simulink model "OSWEC"  (R2021b)
settings: Solver=ode45  StartTime=0  StopTime=200  FixedStep=0.01  MaxStep=0.01  RelTol=1e-3  EnableMultiTasking=on
values from neighbouring files (symbols this model uses):
  N = 25    [PI_reg_nocodesign.mat]
  ptosim = ptoSimClass('Non-Compressible Fluid Hydraulic')    [wecSimInputFile.m]
undefined symbols (not defined in the file or in its folder): body, constraint, geometry, hydroData, pto, X, Y, Z
libraries: nesl_utility x8, sm_lib x7, WECSim_Lib_Body_Elements x2, WECSim_Lib_Constraints x1, WECSim_Lib_Frames x1, PTOSim_Lib x1
settings Model: Creator=mlawson  LastModifiedBy=jackson
settings SolverCC: ZeroCrossControl=DisableAll  AlgebraicLoopSolver=LineSearch  AutoInsertRateTranBlk=on
settings DataIOCC: SaveFormat=Array  SaveOutput=off  SaveTime=off  ReturnWorkspaceOutputs=off
settings OptimizationCC: LifeSpan=inf  SimCompilerOptimization=on
settings DebuggingCC: UnderspecifiedInitializationDetection=Classic  MergeDetectMultiDrivingBlocksExec=none  SolverPrmCheckMsg=warning  AllowSymbolicDim=off  StateNameClashWarn=warning  SFUnexpectedBacktrackingDiag=warning  SFNoUnconditionalDefaultTransitionDiag=warning  SFExecutionAtInitializationDiag=none  SFMachineParentedDataDiag=warning  ArithmeticOperatorsInVariantConditions=warning
settings HardwareCC: ProdBitPerPointer=32  ProdBitPerSizeT=32  ProdBitPerPtrDiffT=32  ProdLargestAtomicFloat=None  ProdIntDivRoundTo=Undefined  ProdEndianess=Unspecified  ProdWordSize=32  ProdHWDeviceType=32-bit Generic
settings ModelReferenceCC: PropagateSignalLabelsOutOfModel=off
settings SFSimCC: SimUseLocalCustomCode=off  CustomCodeUndefinedFunction=UseInterfaceOnly
settings RTWCC: RTWUseLocalCustomCode=off
settings CodeAppCC: StateflowObjectComments=on
settings GRTTargetCC: TargetLangStandard=C89/C90 (ANSI)
settings ConfigComp: CovMetricSettings=dw  CovSaveCumulativeToWorkspaceVar=on  CovSaveSingleToWorkspaceVar=on  CovExternalEMLEnable=off  CovSFcnEnable=off
settings SimscapeCC: SimscapeNormalizeSystem=off
settings ConfigurationSet: Description=SimMechanics 2G
settings ExplorerConfigSet: SimMechanicsOpenEditorOnUpdate=off  InternalSimMechanicsExplorerSettings="<ExplorerConfiguration><canonicalview>default</canonicalview><TilePanel><TileInfo><Tiles Columns=\"1\" Count=\"1\" Rows=\"1\"><Column Left=\"2\" Weight=\"1\"/><Column Left=\"1335\"/><Row Top=\"2\" Weight=\"1\"/><Row Top=\"911\"/><Tile Height=\"1\" Width=\"1\" X=\"0\" Y=\"0\"/></Tiles></TileInfo><SceneInfo><SceneViewer><BGColor><R>0.60000002384185791</R><G>0.60000002384185791</G><B>0.60000002384185791</B></BGColor><Camera><Position><X>365.37645888990272</X><Y>-369.82486814446582</Y><Z>359.64809521743916</Z></Position><Center><X>-6.7351450971904585</X><Y>2.2867358426280204</Y><Z>-12.463508769654169</Z></Center><Up><X>-0.40824829046386307</X><Y>0.40824829046386307</Y><Z>0.81649658092772615</Z></Up><Left>-57.820127362122818</Left><Right>57.820127362122818</Right><Bottom>-38.308817187253304</Bottom><Top>38.308817187253304</Top></Camera></SceneViewer></SceneInfo></TilePanel></ExplorerConfiguration>"

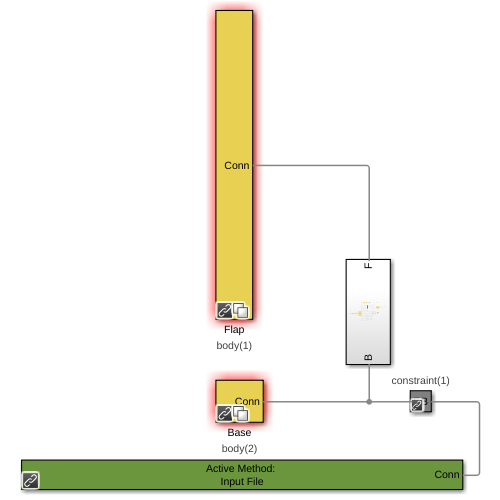
[thumbnail: Simulink's stored preview of the top-level diagram]
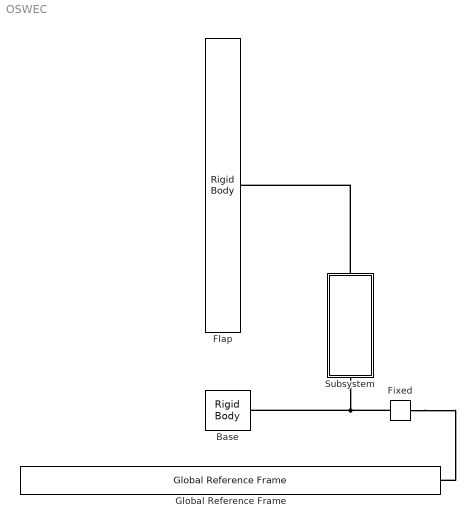
== system OSWEC ==
  Base : WECSim_Lib_Body_Elements/Rigid Body  body=body(2)  h5File=hydroData/*.h5  geometryFile=geometry/*.stl  mass=0  momOfInertia=0 0 0  nhBody=0  nlHydro=0  cg=0 0 0  cb=0 0 0  dof=6  dispVol=0  initLinDisp=0 0 0  initAngularDispAxis=0 1 0  initAngularDispAngle=0  option=0  cd=0 0 0  ca=0 0 0  characteristicArea=0 0 0  VME=0  rgME=0 0 0  z=0 0 1
      settings: SourceProductName=WEC-Sim
  Fixed : WECSim_Lib_Constraints/Fixed  constraint=constraint(1)  loc="0  0  0"  initLinDisp=0 0 0  y=0 1 0  z=0 0 1  upperLimitSpecify=off  upperLimitBound=0  upperLimitTransitionRegionWidth=0  upperLimitStiffness=0  upperLimitDamping=0  lowerLimitSpecify=off  lowerLimitBound=0  lowerLimitTransitionRegionWidth=0  lowerLimitStiffness=0  lowerLimitDamping=0
      settings: AttributesFormatString=%<constraint>  SourceProductName=WEC-Sim
  Flap : WECSim_Lib_Body_Elements/Rigid Body  body=body(1)  h5File=hydroData/*.h5  geometryFile=geometry/*.stl  mass=0  momOfInertia=0 0 0  nhBody=0  nlHydro=0  cg=0 0 0  cb=0 0 0  dof=6  dispVol=0  initLinDisp=0 0 0  initAngularDispAxis=0 1 0  initAngularDispAngle=0  option=0  cd=0 0 0  ca=0 0 0  characteristicArea=0 0 0  VME=0  rgME=0 0 0  z=0 0 1
      settings: SourceProductName=WEC-Sim
  Global Reference Frame : WECSim_Lib_Frames/Global Reference Frame  waves=waves  simu=simu  ParamInput=Input File  InputFile=wecSimInputFile.m  mode=normal  explorer=off  solver=ode4  startTime=0  rampTime=100  endTime=400  dt=0.1  CITime=60  ssCalc=0  WaveClass=regular  H=2.5  T=8  etaDataFile=NOT DEFINED  spectrumDataFile=NOT DEFINED  waveDir=0  waveSpread=1  spectrumType=NOT DEFINED  freqDisc=EqualEnergy  phaseSeed=0
      settings: SourceProductName=WEC-Sim
  Subsystem : Subsystem
  connections:
  Fixed/LConn1 -- Global Reference Frame/RConn1
  Fixed/RConn1 -- Base/RConn1 -- Subsystem/LConn1
  Subsystem/RConn1 -- Flap/RConn1

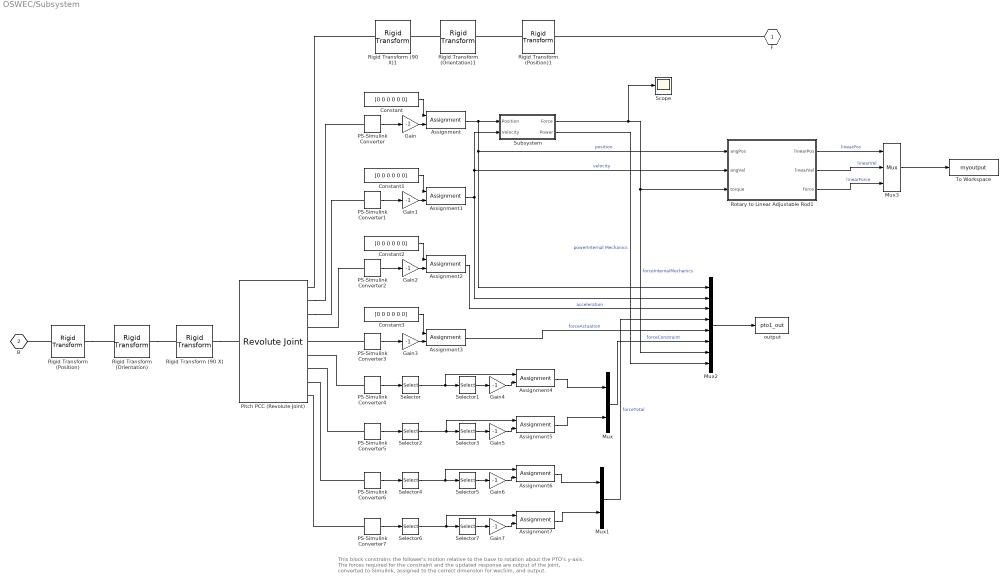
== system OSWEC/Subsystem ==
  note: This block constrains the follower's motion relative to the base to rotation about the PTO's y-axis. The forces required for the constraint and the updated response are output of the joint, converted to Simulink, assigned to the correct dimension for wecSim, and output.
  "Assignment " : Assignment  IndexOptions=Index vector (dialog)  Indices=5  OutputSizes=1
  Assignment1 : Assignment  IndexOptions=Index vector (dialog)  Indices=5  OutputSizes=1
  Assignment2 : Assignment  IndexOptions=Index vector (dialog)  Indices=5  OutputSizes=1
  Assignment3 : Assignment  IndexOptions=Index vector (dialog)  Indices=5  OutputSizes=1
  Assignment{4..7} (4 alike) : Assignment  DiagnosticForDimensions=Warning  IndexOptions=Index vector (dialog)  Indices=2  OutputSizes=1
  Constant{,1..3} (4 alike) : Constant  Value=[0 0 0 0 0 0]
  Gain{,1..7} (8 alike) : Gain  Gain=-1
  Mux : Mux  Inputs=2
  Mux1 : Mux  Inputs=2
  Mux2 : Mux  Inputs=8
  Mux3 : Mux  Inputs=3
  PS-Simulink Converter{,1..7} (8 alike) : nesl_utility/PS-Simulink Converter  PhysicalDomain=network_engine_domain  SubClassName=ps_output  LeftPortType=input  RightPortType=output  PseudoPeriodic=off  Frequencies=[]  Unit=1  AffineConversion=off
      settings: SourceProductBaseCode=PW,SS
  Pitch PCC (Revolute Joint) : sm_lib/Joints/Revolute Joint  JointMode=Normal  SenseConstraintForce=on  SenseConstraintForceX=off  SenseConstraintForceY=off  SenseConstraintForceZ=off  SenseConstraintTorque=on  SenseConstraintTorqueX=off  SenseConstraintTorqueY=off  SenseConstraintTorqueZ=off  SenseTotalForce=on  SenseTotalForceX=off  SenseTotalForceY=off  SenseTotalForceZ=off  SenseTotalTorque=on  SenseTotalTorqueX=off  SenseTotalTorqueY=off  SenseTotalTorqueZ=off  CompositeWrenchDir=BaseOnFollower  CompositeWrenchFrame=BaseFrame  EquilibriumPosition=pto.equilibriumPosition  EquilibriumPositionUnits=deg  SpringStiffness=pto.k  SpringStiffnessUnits=N*m/rad  DampingCoefficient=pto.c  DampingCoefficientUnits=N*m/(rad/s)  TorqueActuationMode=NoTorque  MotionActuationMode=ComputedMotion  SensePosition=on  SenseVelocity=on  SenseAcceleration=on  SenseTorqueForce=on  SenseLowerLimitTorqueForce=off  SenseUpperLimitTorqueForce=off  LowerLimitSpecify=off  LowerLimitBound=pto.hardStops.lowerLimitBound  LowerLimitBoundUnits=deg  LowerLimitStiffness=pto.hardStops.lowerLimitStiffness  LowerLimitStiffnessUnits=N*m/deg  LowerLimitDamping=pto.hardStops.lowerLimitDamping  LowerLimitDampingUnits=N*m/(deg/s)  LowerLimitTransitionRegionWidth=pto.hardStops.lowerLimitTransitionRegionWidth  LowerLimitTransitionRegionWidthUnits=deg  UpperLimitSpecify=off  UpperLimitBound=pto.hardStops.upperLimitBound  UpperLimitBoundUnits=deg  UpperLimitStiffness=pto.hardStops.upperLimitStiffness  UpperLimitStiffnessUnits=N*m/deg  UpperLimitDamping=pto.hardStops.upperLimitDamping  UpperLimitDampingUnits=N*m/(deg/s)  UpperLimitTransitionRegionWidth=pto.hardStops.upperLimitTransitionRegionWidth  UpperLimitTransitionRegionWidthUnits=deg  PositionTargetSpecify=off  PositionTargetPriority=High  PositionTargetValue=0  PositionTargetValueUnits=deg  VelocityTargetSpecify=off  VelocityTargetPriority=High  VelocityTargetValue=0  VelocityTargetValueUnits=deg/s
  Rigid Transform (Position) : sm_lib/Frames and Transforms/Rigid Transform  TranslationMethod=Cartesian  TranslationStandardOffset=0  TranslationLengthUnit=m  TranslationStandardAxis=+Z  TranslationCartesianOffset=pto.initDisp.initLinDisp + pto.loc  TranslationROffset=0  TranslationROffsetUnits=m  TranslationZOffset=0  TranslationZOffsetUnits=m  TranslationThetaOffset=0  TranslationThetaOffsetUnits=deg  RotationMethod=None  RotationAngleUnits=rad  RotationStandardAxis=+Y  RotationAngle=0  RotationArbitraryAxis=[0 1 0]  FollAlignAxisA=+X  BaseAlignAxisA=+Y  FollAlignAxisB=+Y  BaseAlignAxisB=+Z  RotationSequenceAxes=FollowerAxes  RotationSequence=XYX  RotationSequenceAngles=[0 0 0]  RotationSequenceAnglesUnits=deg  RotationMatrix=[1 0 0; 0 1 0; 0 0 1]
  Rigid Transform (Position)1 : sm_lib/Frames and Transforms/Rigid Transform  TranslationMethod=Cartesian  TranslationStandardOffset=0  TranslationLengthUnit=m  TranslationStandardAxis=+Z  TranslationCartesianOffset=pto.initDisp.initLinDisp + pto.loc  TranslationROffset=0  TranslationROffsetUnits=m  TranslationZOffset=0  TranslationZOffsetUnits=m  TranslationThetaOffset=0  TranslationThetaOffsetUnits=deg  RotationMethod=None  RotationAngleUnits=rad  RotationStandardAxis=+Y  RotationAngle=0  RotationArbitraryAxis=[0 1 0]  FollAlignAxisA=+X  BaseAlignAxisA=+Y  FollAlignAxisB=+Y  BaseAlignAxisB=+Z  RotationSequenceAxes=FollowerAxes  RotationSequence=XYX  RotationSequenceAngles=[0 0 0]  RotationSequenceAnglesUnits=deg  RotationMatrix=[1 0 0; 0 1 0; 0 0 1]
  Rigid Transform (90 X) : sm_lib/Frames and Transforms/Rigid Transform  TranslationMethod=None  TranslationStandardOffset=0  TranslationLengthUnit=m  TranslationStandardAxis=+Z  TranslationCartesianOffset=0  TranslationROffset=0  TranslationROffsetUnits=m  TranslationZOffset=0  TranslationZOffsetUnits=m  TranslationThetaOffset=0  TranslationThetaOffsetUnits=deg  RotationMethod=StandardAxis  RotationAngleUnits=deg  RotationStandardAxis=+X  RotationAngle=90  RotationArbitraryAxis=[0 1 0]  FollAlignAxisA=+X  BaseAlignAxisA=+Y  FollAlignAxisB=+Y  BaseAlignAxisB=+Z  RotationSequenceAxes=FollowerAxes  RotationSequence=XYX  RotationSequenceAngles=[0 0 0]  RotationSequenceAnglesUnits=deg  RotationMatrix=[1 0 0; 0 1 0; 0 0 1]
  Rigid Transform (90 X)1 : sm_lib/Frames and Transforms/Rigid Transform  TranslationMethod=None  TranslationStandardOffset=0  TranslationLengthUnit=m  TranslationStandardAxis=+Z  TranslationCartesianOffset=0  TranslationROffset=0  TranslationROffsetUnits=m  TranslationZOffset=0  TranslationZOffsetUnits=m  TranslationThetaOffset=0  TranslationThetaOffsetUnits=deg  RotationMethod=StandardAxis  RotationAngleUnits=deg  RotationStandardAxis=+X  RotationAngle=90  RotationArbitraryAxis=[0 1 0]  FollAlignAxisA=+X  BaseAlignAxisA=+Y  FollAlignAxisB=+Y  BaseAlignAxisB=+Z  RotationSequenceAxes=FollowerAxes  RotationSequence=XYX  RotationSequenceAngles=[0 0 0]  RotationSequenceAnglesUnits=deg  RotationMatrix=[1 0 0; 0 1 0; 0 0 1]
  Rigid Transform (Orientation) : sm_lib/Frames and Transforms/Rigid Transform  TranslationMethod=None  TranslationStandardOffset=0  TranslationLengthUnit=m  TranslationStandardAxis=+Z  TranslationCartesianOffset=0  TranslationROffset=0  TranslationROffsetUnits=m  TranslationZOffset=0  TranslationZOffsetUnits=m  TranslationThetaOffset=0  TranslationThetaOffsetUnits=deg  RotationMethod=RotationMatrix  RotationAngleUnits=rad  RotationStandardAxis=+Y  RotationAngle=0  RotationArbitraryAxis=[0 1 0]  FollAlignAxisA=+X  BaseAlignAxisA=+Y  FollAlignAxisB=+Y  BaseAlignAxisB=+Z  RotationSequenceAxes=FollowerAxes  RotationSequence=XYX  RotationSequenceAngles=[0 0 0]  RotationSequenceAnglesUnits=deg  RotationMatrix=pto.orientation.rotationMatrix
  Rigid Transform (Orientation)1 : sm_lib/Frames and Transforms/Rigid Transform  TranslationMethod=None  TranslationStandardOffset=0  TranslationLengthUnit=m  TranslationStandardAxis=+Z  TranslationCartesianOffset=0  TranslationROffset=0  TranslationROffsetUnits=m  TranslationZOffset=0  TranslationZOffsetUnits=m  TranslationThetaOffset=0  TranslationThetaOffsetUnits=deg  RotationMethod=RotationMatrix  RotationAngleUnits=rad  RotationStandardAxis=+Y  RotationAngle=0  RotationArbitraryAxis=[0 1 0]  FollAlignAxisA=+X  BaseAlignAxisA=+Y  FollAlignAxisB=+Y  BaseAlignAxisB=+Z  RotationSequenceAxes=FollowerAxes  RotationSequence=XYX  RotationSequenceAngles=[0 0 0]  RotationSequenceAnglesUnits=deg  RotationMatrix=pto.orientation.rotationMatrix
  Rotary to Linear Adjustable Rod1 : Subsystem  AncestorBlock=PTOSim_Lib/Motion Conversion/Rotary to Linear Adjustable Rod  mask{ptosim=ptosim.motionMechanism(1)}
      mask prompts: ptosim "Telescope Name:"
      mask init:
      | % if exist('ptosim','var')
      | %     h = [gcb '/To Workspace'];
      | %     responseName = ['motionMechanism' num2str(ptosim.number) '_out'];
      | %     set_param(h,'VariableName',responseName);
      | %     if ischar(ptosim.crank)==1 ...
      | %             || ischar(ptosim.rodInit)==1 ...
      | %             || ischar(ptosim.offset)==1 ...
      | %             error('One of the rotary to linear adjustable rod variables is undefined. For example, ptosim.motionMechanism.variableName')
      | %     end
      | % end
      | % clear h responseName
  Scope : Scope
  Selector{,2,4,6} (4 alike) : Selector  InputPortWidth=3  IndexOptions=Index vector (dialog)  Indices=[1 3 2]  OutputSizes=1
  Selector{1,3,5,7} (4 alike) : Selector  InputPortWidth=3  IndexOptions=Index vector (dialog)  Indices=[2]  OutputSizes=1
  Subsystem : Subsystem
  To Workspace : ToWorkspace  VariableName=myoutput  SaveFormat=Structure With Time  SampleTime=-1
  output : ToWorkspace  VariableName=pto1_out  SaveFormat=Structure With Time  SampleTime=-1
      settings: Decimation=round(simu.dtOut/simu.dt,0)
  F : PMIOPort  Side=Right
  B : PMIOPort  Port=2  Side=Left
  wires:
  Selector6/1 -> Selector7/1, Assignment7/1
  Gain4/1 -> Assignment4/2
  Selector2/1 -> Assignment5/1, Selector3/1
  Constant2/1 -> Assignment2/1
  PS-Simulink Converter3/1 -> Gain3/1
  Gain6/1 -> Assignment6/2
  Mux1/1 -> Mux2/4  "forceTotal"
  Assignment2/1 -> Mux2/3  "acceleration"
  Assignment3/1 -> Mux2/5  "forceActuation"
  Gain7/1 -> Assignment7/2
  Selector1/1 -> Gain4/1
  Gain3/1 -> Assignment3/2
  Gain/1 -> "Assignment "/2
  Selector7/1 -> Gain7/1
  PS-Simulink Converter/1 -> Gain/1
  Gain5/1 -> Assignment5/2
  Assignment6/1 -> Mux1/1
  Subsystem/2(Power) -> Mux2/8  "powerInternal Mechanics"
  Assignment7/1 -> Mux1/2
  PS-Simulink Converter6/1 -> Selector4/1
  Assignment1/1 -> Mux2/2, Subsystem/2(Velocity), Rotary to Linear Adjustable Rod1/2(angVel)  "velocity"
  Gain2/1 -> Assignment2/2
  Subsystem/1(Force) -> Scope/1, Rotary to Linear Adjustable Rod1/3(torque), Mux2/7  "forceInternalMechanics"
  Constant3/1 -> Assignment3/1
  PS-Simulink Converter7/1 -> Selector6/1
  Mux2/1 -> output/1
  PS-Simulink Converter4/1 -> Selector/1
  Gain1/1 -> Assignment1/2
  Selector5/1 -> Gain6/1
  Mux/1 -> Mux2/6  "forceConstraint"
  Constant1/1 -> Assignment1/1
  Assignment4/1 -> Mux/1
  "Assignment "/1 -> Rotary to Linear Adjustable Rod1/1(angPos), Mux2/1, Subsystem/1(Position)  "position"
  Selector4/1 -> Selector5/1, Assignment6/1
  PS-Simulink Converter1/1 -> Gain1/1
  Assignment5/1 -> Mux/2
  PS-Simulink Converter5/1 -> Selector2/1
  Selector3/1 -> Gain5/1
  PS-Simulink Converter2/1 -> Gain2/1
  Selector/1 -> Assignment4/1, Selector1/1
  Constant/1 -> "Assignment "/1
  Rotary to Linear Adjustable Rod1/1(linearPos) -> Mux3/1  "linearPos"
  Rotary to Linear Adjustable Rod1/2(linearVel) -> Mux3/2  "linearVel"
  Rotary to Linear Adjustable Rod1/3(force) -> Mux3/3  "linearForce"
  Mux3/1 -> To Workspace/1
  connections:
  Rigid Transform (Orientation)1/RConn1 -- Rigid Transform (90 X)1/LConn1
  PS-Simulink Converter5/LConn1 -- Pitch PCC (Revolute Joint)/RConn7
  Rigid Transform (Position)1/RConn1 -- Rigid Transform (Orientation)1/LConn1
  PS-Simulink Converter7/LConn1 -- Pitch PCC (Revolute Joint)/RConn9
  F/RConn1 -- Rigid Transform (Position)1/LConn1
  Pitch PCC (Revolute Joint)/RConn2 -- PS-Simulink Converter/LConn1
  PS-Simulink Converter4/LConn1 -- Pitch PCC (Revolute Joint)/RConn6
  PS-Simulink Converter6/LConn1 -- Pitch PCC (Revolute Joint)/RConn8
  Rigid Transform (Position)/RConn1 -- Rigid Transform (Orientation)/LConn1
  Rigid Transform (Orientation)/RConn1 -- Rigid Transform (90 X)/LConn1
  PS-Simulink Converter3/LConn1 -- Pitch PCC (Revolute Joint)/RConn5
  Rigid Transform (Position)/LConn1 -- B/RConn1
  PS-Simulink Converter2/LConn1 -- Pitch PCC (Revolute Joint)/RConn4
  Rigid Transform (90 X)1/RConn1 -- Pitch PCC (Revolute Joint)/RConn1
  Rigid Transform (90 X)/RConn1 -- Pitch PCC (Revolute Joint)/LConn1
  Pitch PCC (Revolute Joint)/RConn3 -- PS-Simulink Converter1/LConn1

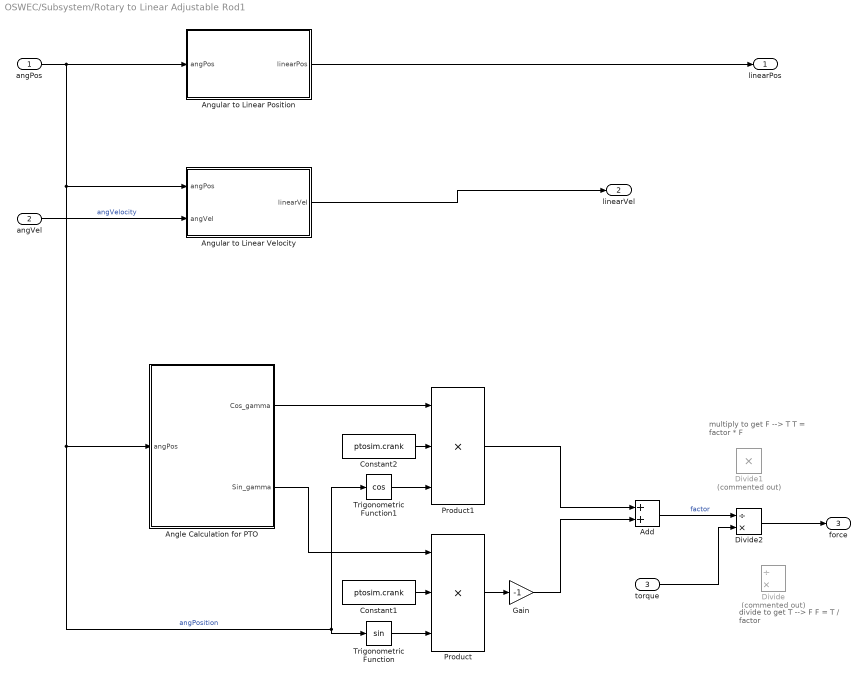
== system OSWEC/Subsystem/Rotary to Linear Adjustable Rod1 ==
  note: multiply to get F --> T
      | T = factor * F
  note: divide to get T --> F
      | F = T / factor
  angPos : Inport
  angVel : Inport  Port=2
  torque : Inport  Port=3
  Add : Sum
  Angle Calculation for PTO : Subsystem
  Angular to Linear Position : Subsystem
  Angular to Linear Velocity : Subsystem
  Constant1 : Constant  Value=ptosim.crank
  Constant2 : Constant  Value=ptosim.crank
  Divide : Product  Commented=on  Inputs=/*
  Divide1 : Product  Commented=on  Inputs=**
  Divide2 : Product  Inputs=/*
  Gain : Gain  Gain=-1
  Product : Product  Inputs=3
  Product1 : Product  Inputs=3
  Trigonometric Function : Trigonometry
  Trigonometric Function1 : Trigonometry  Operator=cos
  linearPos : Outport
  linearVel : Outport  Port=2
  force : Outport  Port=3
  wires:
  Product/1 -> Gain/1
  Constant1/1 -> Product/2
  Trigonometric Function/1 -> Product/3
  Constant2/1 -> Product1/2
  Angle Calculation for PTO/1(Cos_gamma) -> Product1/1
  Trigonometric Function1/1 -> Product1/3
  Angle Calculation for PTO/2(Sin_gamma) -> Product/1
  Gain/1 -> Add/2
  Product1/1 -> Add/1
  angPos/1 -> Angular to Linear Position/1(angPos), Trigonometric Function1/1, Trigonometric Function/1, Angle Calculation for PTO/1(angPos), Angular to Linear Velocity/1(angPos)  "angPosition"
  Angular to Linear Velocity/1(linearVel) -> linearVel/1
  angVel/1 -> Angular to Linear Velocity/2(angVel)  "angVelocity"
  Angular to Linear Position/1(linearPos) -> linearPos/1
  Divide2/1 -> force/1
  Add/1 -> Divide2/1  "factor"
  torque/1 -> Divide2/2

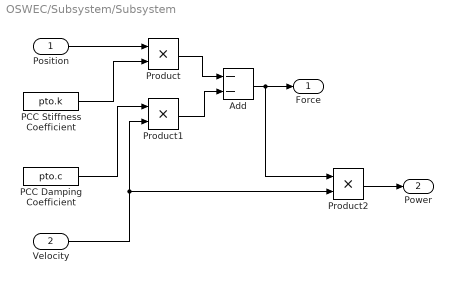
== system OSWEC/Subsystem/Subsystem ==
  Position : Inport
  Velocity : Inport  Port=2
  Add : Sum  Inputs=--
  PCC Damping Coefficient : Constant  Value=pto.c
  PCC Stiffness Coefficient : Constant  Value=pto.k
  Product : Product  Inputs=**
  Product1 : Product  Inputs=**
  Product2 : Product  Inputs=**
  Force : Outport
  Power : Outport  Port=2
  wires:
  PCC Damping Coefficient/1 -> Product1/1
  Velocity/1 -> Product2/2, Product1/2
  Position/1 -> Product/1
  Product2/1 -> Power/1
  PCC Stiffness Coefficient/1 -> Product/2
  Product/1 -> Add/1
  Product1/1 -> Add/2
  Add/1 -> Product2/1, Force/1

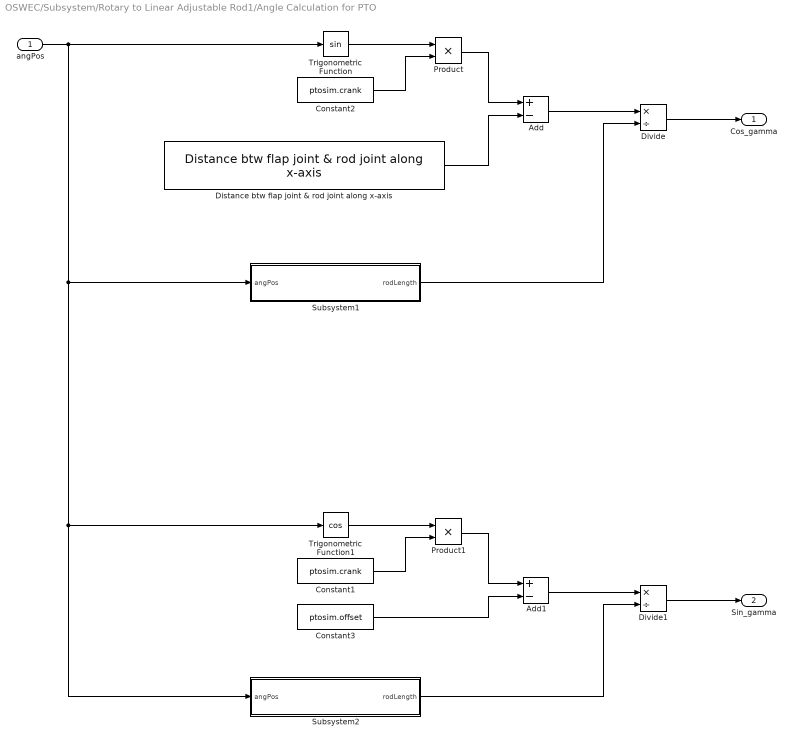
== system OSWEC/Subsystem/Rotary to Linear Adjustable Rod1/Angle Calculation for PTO ==
  angPos : Inport
  Add : Sum  Inputs=+-
  Add1 : Sum  Inputs=+-
  Constant1 : Constant  Value=ptosim.crank
  Constant2 : Constant  Value=ptosim.crank
  Constant3 : Constant  Value=ptosim.offset
  Distance btw flap joint & rod joint along x-axis : PTOSim_Lib/Motion Conversion/Rotary to Linear Adjustable Rod/Angular to Linear Velocity/Subsystem/Distance btw flap joint & rod joint along x-axis  SystemSampleTime=-1  VariantActivationTime=update diagram  Latency=0  AutoFrameSizeCalculation=off
      settings: SourceProductName=PTO-Sim
  Divide : Product  Inputs=*/
  Divide1 : Product  Inputs=*/
  Product : Product
  Product1 : Product
  Subsystem1 : Subsystem  AncestorBlock=|
      | PTOSim_Lib/Motion Conversion/Rotary to Linear
      | Adjustable Rod/Angular to Linear
      | Velocity/Subsystem
  Subsystem2 : Subsystem  AncestorBlock=|
      | PTOSim_Lib/Motion Conversion/Rotary to Linear
      | Adjustable Rod/Angular to Linear
      | Velocity/Subsystem
  Trigonometric Function : Trigonometry
  Trigonometric Function1 : Trigonometry  Operator=cos
  Cos_gamma : Outport
  Sin_gamma : Outport  Port=2
  wires:
  Divide1/1 -> Sin_gamma/1
  angPos/1 -> Trigonometric Function/1, Trigonometric Function1/1, Subsystem2/1(angPos), Subsystem1/1(angPos)
  Add1/1 -> Divide1/1
  Constant3/1 -> Add1/2
  Product1/1 -> Add1/1
  Constant1/1 -> Product1/2
  Trigonometric Function1/1 -> Product1/1
  Subsystem2/1(rodLength) -> Divide1/2
  Divide/1 -> Cos_gamma/1
  Subsystem1/1(rodLength) -> Divide/2
  Add/1 -> Divide/1
  Constant2/1 -> Product/2
  Distance btw flap joint & rod joint along x-axis/1 -> Add/2
  Product/1 -> Add/1
  Trigonometric Function/1 -> Product/1

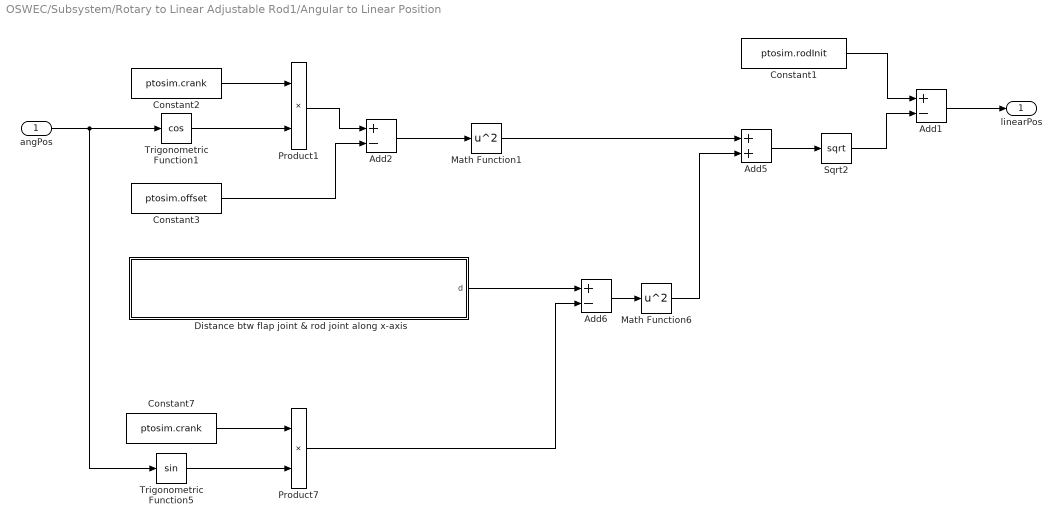
== system OSWEC/Subsystem/Rotary to Linear Adjustable Rod1/Angular to Linear Position ==
  angPos : Inport
  Add1 : Sum  Inputs=+-
  Add2 : Sum  Inputs=+-
  Add5 : Sum
  Add6 : Sum  Inputs=+-
  Constant1 : Constant  Value=ptosim.rodInit
  Constant2 : Constant  Value=ptosim.crank
  Constant3 : Constant  Value=ptosim.offset
  Constant7 : Constant  Value=ptosim.crank
  Distance btw flap joint & rod joint along x-axis : Subsystem
  Math Function1 : Math  Operator=square  SignedPower=on  SaturateOnIntegerOverflow=on
  Math Function6 : Math  Operator=square  SignedPower=on  SaturateOnIntegerOverflow=on
  Product1 : Product  Inputs=**
  Product7 : Product  Inputs=**
  Sqrt2 : Sqrt  SaturateOnIntegerOverflow=on
  Trigonometric Function1 : Trigonometry  Operator=cos
  Trigonometric Function5 : Trigonometry
  linearPos : Outport
  wires:
  Distance btw flap joint & rod joint along x-axis/1(d) -> Add6/1
  Constant7/1 -> Product7/1
  Math Function1/1 -> Add5/1
  Constant3/1 -> Add2/2
  Product1/1 -> Add2/1
  Trigonometric Function1/1 -> Product1/2
  Constant2/1 -> Product1/1
  Constant1/1 -> Add1/1
  Sqrt2/1 -> Add1/2
  Add5/1 -> Sqrt2/1
  Math Function6/1 -> Add5/2
  Add6/1 -> Math Function6/1
  Product7/1 -> Add6/2
  Trigonometric Function5/1 -> Product7/2
  Add2/1 -> Math Function1/1
  Add1/1 -> linearPos/1
  angPos/1 -> Trigonometric Function1/1, Trigonometric Function5/1

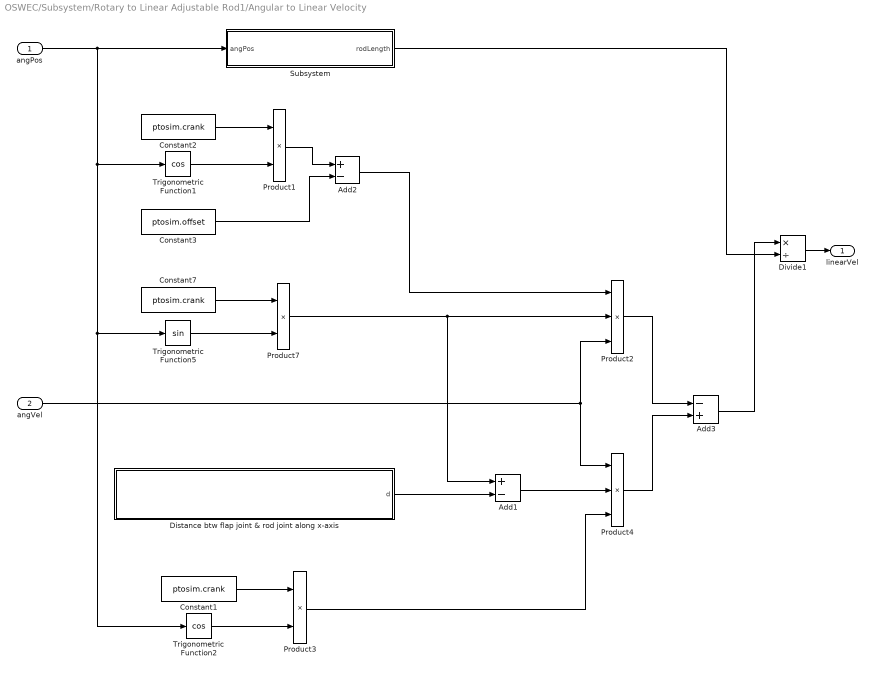
== system OSWEC/Subsystem/Rotary to Linear Adjustable Rod1/Angular to Linear Velocity ==
  angPos : Inport
  angVel : Inport  Port=2
  Add1 : Sum  Inputs=+-
  Add2 : Sum  Inputs=+-
  Add3 : Sum  Inputs=-+
  Constant1 : Constant  Value=ptosim.crank
  Constant2 : Constant  Value=ptosim.crank
  Constant3 : Constant  Value=ptosim.offset
  Constant7 : Constant  Value=ptosim.crank
  Distance btw flap joint & rod joint along x-axis : Subsystem
  Divide1 : Product  Inputs=*/
  Product1 : Product  Inputs=**
  Product2 : Product  Inputs=***
  Product3 : Product  Inputs=**
  Product4 : Product  Inputs=***
  Product7 : Product  Inputs=**
  Subsystem : Subsystem
  Trigonometric Function1 : Trigonometry  Operator=cos
  Trigonometric Function2 : Trigonometry  Operator=cos
  Trigonometric Function5 : Trigonometry
  linearVel : Outport
  wires:
  Divide1/1 -> linearVel/1
  Add3/1 -> Divide1/1
  Product4/1 -> Add3/2
  Product2/1 -> Add3/1
  Subsystem/1(rodLength) -> Divide1/2
  Add1/1 -> Product4/2
  angPos/1 -> Subsystem/1(angPos), Trigonometric Function1/1, Trigonometric Function2/1, Trigonometric Function5/1
  Product3/1 -> Product4/3
  Trigonometric Function2/1 -> Product3/2
  Constant1/1 -> Product3/1
  Distance btw flap joint & rod joint along x-axis/1(d) -> Add1/2
  angVel/1 -> Product4/1, Product2/3
  Constant7/1 -> Product7/1
  Product7/1 -> Product2/2, Add1/1
  Trigonometric Function5/1 -> Product7/2
  Constant3/1 -> Add2/2
  Product1/1 -> Add2/1
  Trigonometric Function1/1 -> Product1/2
  Constant2/1 -> Product1/1
  Add2/1 -> Product2/1

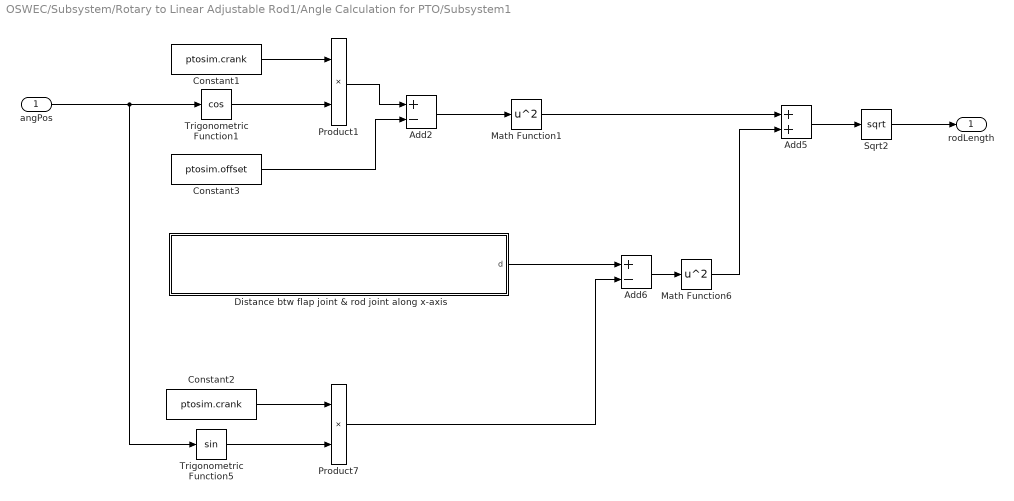
== system OSWEC/Subsystem/Rotary to Linear Adjustable Rod1/Angle Calculation for PTO/Subsystem1 ==
  angPos : Inport
  Add2 : Sum  Inputs=+-
  Add5 : Sum
  Add6 : Sum  Inputs=+-
  Constant1 : Constant  Value=ptosim.crank
  Constant2 : Constant  Value=ptosim.crank
  Constant3 : Constant  Value=ptosim.offset
  Distance btw flap joint & rod joint along x-axis : Subsystem
  Math Function1 : Math  Operator=square  SignedPower=on  SaturateOnIntegerOverflow=on
  Math Function6 : Math  Operator=square  SignedPower=on  SaturateOnIntegerOverflow=on
  Product1 : Product  Inputs=**
  Product7 : Product  Inputs=**
  Sqrt2 : Sqrt  SaturateOnIntegerOverflow=on
  Trigonometric Function1 : Trigonometry  Operator=cos
  Trigonometric Function5 : Trigonometry
  rodLength : Outport
  wires:
  angPos/1 -> Trigonometric Function5/1, Trigonometric Function1/1
  Add2/1 -> Math Function1/1
  Trigonometric Function5/1 -> Product7/2
  Product7/1 -> Add6/2
  Add6/1 -> Math Function6/1
  Math Function6/1 -> Add5/2
  Add5/1 -> Sqrt2/1
  Sqrt2/1 -> rodLength/1
  Constant1/1 -> Product1/1
  Trigonometric Function1/1 -> Product1/2
  Product1/1 -> Add2/1
  Constant3/1 -> Add2/2
  Math Function1/1 -> Add5/1
  Constant2/1 -> Product7/1
  Distance btw flap joint & rod joint along x-axis/1(d) -> Add6/1

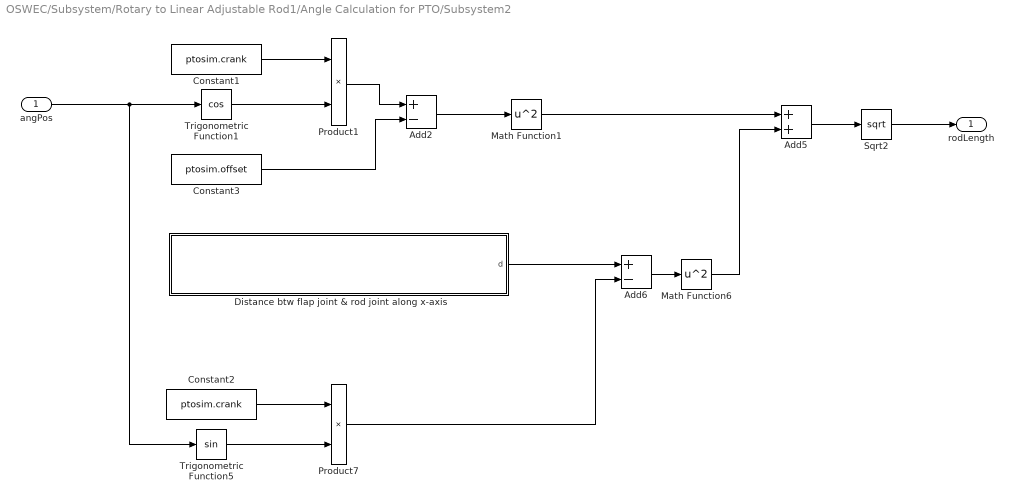
== system OSWEC/Subsystem/Rotary to Linear Adjustable Rod1/Angle Calculation for PTO/Subsystem2 ==
  angPos : Inport
  Add2 : Sum  Inputs=+-
  Add5 : Sum
  Add6 : Sum  Inputs=+-
  Constant1 : Constant  Value=ptosim.crank
  Constant2 : Constant  Value=ptosim.crank
  Constant3 : Constant  Value=ptosim.offset
  Distance btw flap joint & rod joint along x-axis : Subsystem
  Math Function1 : Math  Operator=square  SignedPower=on  SaturateOnIntegerOverflow=on
  Math Function6 : Math  Operator=square  SignedPower=on  SaturateOnIntegerOverflow=on
  Product1 : Product  Inputs=**
  Product7 : Product  Inputs=**
  Sqrt2 : Sqrt  SaturateOnIntegerOverflow=on
  Trigonometric Function1 : Trigonometry  Operator=cos
  Trigonometric Function5 : Trigonometry
  rodLength : Outport
  wires:
  angPos/1 -> Trigonometric Function5/1, Trigonometric Function1/1
  Add2/1 -> Math Function1/1
  Trigonometric Function5/1 -> Product7/2
  Product7/1 -> Add6/2
  Add6/1 -> Math Function6/1
  Math Function6/1 -> Add5/2
  Add5/1 -> Sqrt2/1
  Sqrt2/1 -> rodLength/1
  Constant1/1 -> Product1/1
  Trigonometric Function1/1 -> Product1/2
  Product1/1 -> Add2/1
  Constant3/1 -> Add2/2
  Math Function1/1 -> Add5/1
  Constant2/1 -> Product7/1
  Distance btw flap joint & rod joint along x-axis/1(d) -> Add6/1

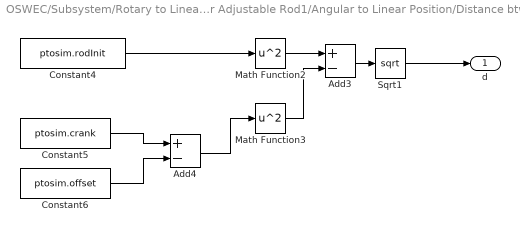
== system OSWEC/Subsystem/Rotary to Linear Adjustable Rod1/Angular to Linear Position/Distance btw flap joint & rod joint along x-axis ==
  Add3 : Sum  Inputs=+-
  Add4 : Sum  Inputs=+-
  Constant4 : Constant  Value=ptosim.rodInit
  Constant5 : Constant  Value=ptosim.crank
  Constant6 : Constant  Value=ptosim.offset
  Math Function2 : Math  Operator=square  SignedPower=on  SaturateOnIntegerOverflow=on
  Math Function3 : Math  Operator=square  SignedPower=on  SaturateOnIntegerOverflow=on
  Sqrt1 : Sqrt  SaturateOnIntegerOverflow=on
  d : Outport
  wires:
  Sqrt1/1 -> d/1
  Math Function2/1 -> Add3/1
  Math Function3/1 -> Add3/2
  Add4/1 -> Math Function3/1
  Constant6/1 -> Add4/2
  Constant5/1 -> Add4/1
  Constant4/1 -> Math Function2/1
  Add3/1 -> Sqrt1/1

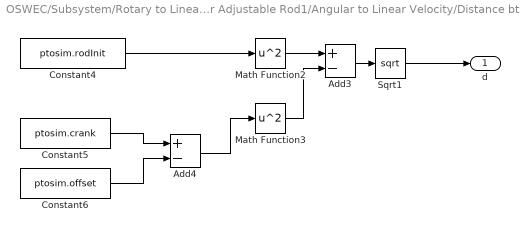
== system OSWEC/Subsystem/Rotary to Linear Adjustable Rod1/Angular to Linear Velocity/Distance btw flap joint & rod joint along x-axis ==
  Add3 : Sum  Inputs=+-
  Add4 : Sum  Inputs=+-
  Constant4 : Constant  Value=ptosim.rodInit
  Constant5 : Constant  Value=ptosim.crank
  Constant6 : Constant  Value=ptosim.offset
  Math Function2 : Math  Operator=square  SignedPower=on  SaturateOnIntegerOverflow=on
  Math Function3 : Math  Operator=square  SignedPower=on  SaturateOnIntegerOverflow=on
  Sqrt1 : Sqrt  SaturateOnIntegerOverflow=on
  d : Outport
  wires:
  Sqrt1/1 -> d/1
  Math Function2/1 -> Add3/1
  Math Function3/1 -> Add3/2
  Add4/1 -> Math Function3/1
  Constant6/1 -> Add4/2
  Constant5/1 -> Add4/1
  Constant4/1 -> Math Function2/1
  Add3/1 -> Sqrt1/1

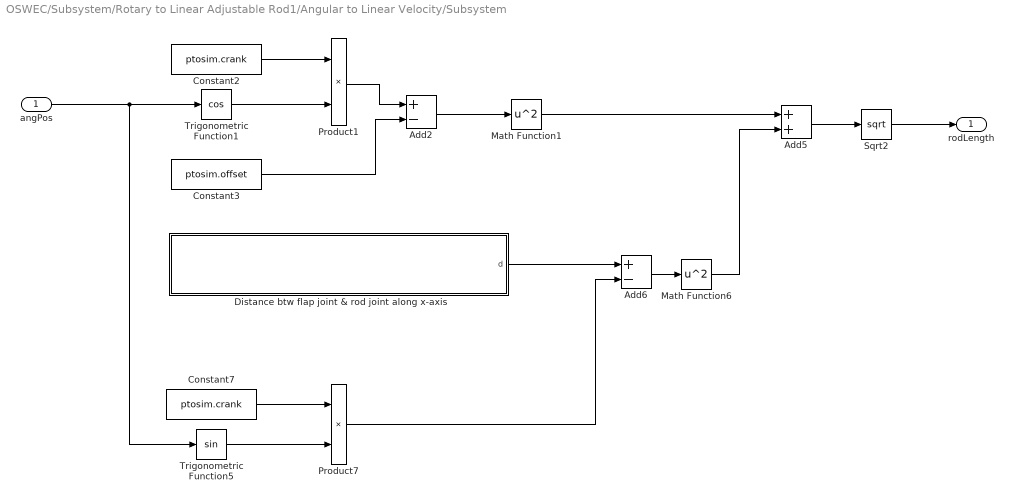
== system OSWEC/Subsystem/Rotary to Linear Adjustable Rod1/Angular to Linear Velocity/Subsystem ==
  angPos : Inport
  Add2 : Sum  Inputs=+-
  Add5 : Sum
  Add6 : Sum  Inputs=+-
  Constant2 : Constant  Value=ptosim.crank
  Constant3 : Constant  Value=ptosim.offset
  Constant7 : Constant  Value=ptosim.crank
  Distance btw flap joint & rod joint along x-axis : Subsystem
  Math Function1 : Math  Operator=square  SignedPower=on  SaturateOnIntegerOverflow=on
  Math Function6 : Math  Operator=square  SignedPower=on  SaturateOnIntegerOverflow=on
  Product1 : Product  Inputs=**
  Product7 : Product  Inputs=**
  Sqrt2 : Sqrt  SaturateOnIntegerOverflow=on
  Trigonometric Function1 : Trigonometry  Operator=cos
  Trigonometric Function5 : Trigonometry
  rodLength : Outport
  wires:
  Distance btw flap joint & rod joint along x-axis/1(d) -> Add6/1
  Constant7/1 -> Product7/1
  Math Function1/1 -> Add5/1
  Constant3/1 -> Add2/2
  Product1/1 -> Add2/1
  Trigonometric Function1/1 -> Product1/2
  Constant2/1 -> Product1/1
  Sqrt2/1 -> rodLength/1
  Add5/1 -> Sqrt2/1
  Math Function6/1 -> Add5/2
  Add6/1 -> Math Function6/1
  Product7/1 -> Add6/2
  Trigonometric Function5/1 -> Product7/2
  Add2/1 -> Math Function1/1
  angPos/1 -> Trigonometric Function1/1, Trigonometric Function5/1

== system OSWEC/Subsystem/Rotary to Linear Adjustable Rod1/Angle Calculation for PTO/Subsystem1/Distance btw flap joint & rod joint along x-axis ==
  Add3 : Sum  Inputs=+-
  Add4 : Sum  Inputs=+-
  Constant1 : Constant  Value=ptosim.crank
  Constant2 : Constant  Value=ptosim.rodInit
  Constant3 : Constant  Value=ptosim.offset
  Math Function2 : Math  Operator=square  SignedPower=on  SaturateOnIntegerOverflow=on
  Math Function3 : Math  Operator=square  SignedPower=on  SaturateOnIntegerOverflow=on
  Sqrt1 : Sqrt  SaturateOnIntegerOverflow=on
  d : Outport
  wires:
  Add3/1 -> Sqrt1/1
  Constant2/1 -> Math Function2/1
  Constant1/1 -> Add4/1
  Constant3/1 -> Add4/2
  Add4/1 -> Math Function3/1
  Math Function3/1 -> Add3/2
  Math Function2/1 -> Add3/1
  Sqrt1/1 -> d/1

== system OSWEC/Subsystem/Rotary to Linear Adjustable Rod1/Angle Calculation for PTO/Subsystem2/Distance btw flap joint & rod joint along x-axis ==
  Add3 : Sum  Inputs=+-
  Add4 : Sum  Inputs=+-
  Constant1 : Constant  Value=ptosim.crank
  Constant2 : Constant  Value=ptosim.rodInit
  Constant3 : Constant  Value=ptosim.offset
  Math Function2 : Math  Operator=square  SignedPower=on  SaturateOnIntegerOverflow=on
  Math Function3 : Math  Operator=square  SignedPower=on  SaturateOnIntegerOverflow=on
  Sqrt1 : Sqrt  SaturateOnIntegerOverflow=on
  d : Outport
  wires:
  Add3/1 -> Sqrt1/1
  Constant2/1 -> Math Function2/1
  Constant1/1 -> Add4/1
  Constant3/1 -> Add4/2
  Add4/1 -> Math Function3/1
  Math Function3/1 -> Add3/2
  Math Function2/1 -> Add3/1
  Sqrt1/1 -> d/1

== system OSWEC/Subsystem/Rotary to Linear Adjustable Rod1/Angular to Linear Velocity/Subsystem/Distance btw flap joint & rod joint along x-axis ==
  Add3 : Sum  Inputs=+-
  Add4 : Sum  Inputs=+-
  Constant4 : Constant  Value=ptosim.rodInit
  Constant5 : Constant  Value=ptosim.crank
  Constant6 : Constant  Value=ptosim.offset
  Math Function2 : Math  Operator=square  SignedPower=on  SaturateOnIntegerOverflow=on
  Math Function3 : Math  Operator=square  SignedPower=on  SaturateOnIntegerOverflow=on
  Sqrt1 : Sqrt  SaturateOnIntegerOverflow=on
  d : Outport
  wires:
  Sqrt1/1 -> d/1
  Math Function2/1 -> Add3/1
  Math Function3/1 -> Add3/2
  Add4/1 -> Math Function3/1
  Constant6/1 -> Add4/2
  Constant5/1 -> Add4/1
  Constant4/1 -> Math Function2/1
  Add3/1 -> Sqrt1/1
